simulink model "assign3q2"  (Simulink 7.4)
settings: Solver=ode23  StartTime=0.0  StopTime=400  RelTol=1e-3
settings Model: Creator=Owner  LastModifiedBy=Owner
settings DataIOCC: LimitDataPoints=off

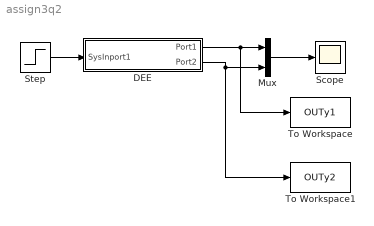
== system assign3q2 ==
  DEE : Subsystem
      settings: OpenFcn=diffeqed
      mask Type: Differential Equation Editor (DEE)
      mask Display: disp('Differential Equation\n Editor')
  Mux : Mux  Inputs=2
  Scope : Scope
  Step : Step  SampleTime=0
  To Workspace : ToWorkspace  VariableName=OUTy1  SampleTime=-1  SaveFormat=Structure
  To Workspace1 : ToWorkspace  VariableName=OUTy2  SampleTime=-1  SaveFormat=Structure
  wires:
  Step/1 -> DEE/1(SysInport1)
  DEE/1(Port1) -> Mux/1, To Workspace/1
  DEE/2(Port2) -> Mux/2, To Workspace1/1
  Mux/1 -> Scope/1

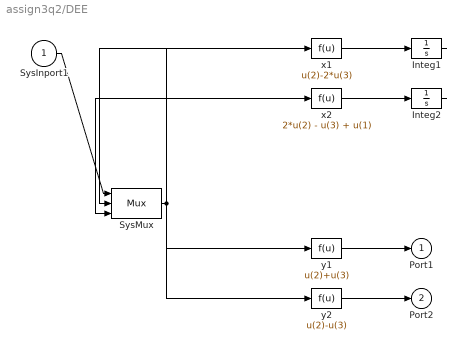
== system assign3q2/DEE ==
  SysInport1 : Inport
  Integ1 : Integrator
  Integ2 : Integrator
  SysMux : Mux  Inputs=3
  x1 : Fcn  Expr=u(2)-2*u(3)
  x2 : Fcn  Expr=2*u(2) - u(3) + u(1)
  y1 : Fcn  Expr=u(2)+u(3)
  y2 : Fcn  Expr=u(2)-u(3)
  Port1 : Outport
  Port2 : Outport  Port=2
  wires:
  SysInport1/1 -> SysMux/1
  SysMux/1 -> x1/1, x2/1, y1/1, y2/1
  x1/1 -> Integ1/1
  Integ1/1 -> SysMux/2
  x2/1 -> Integ2/1
  Integ2/1 -> SysMux/3
  y1/1 -> Port1/1
  y2/1 -> Port2/1
